simulink model "antrieb"  (Simulink 7.8)
settings: Solver=ode3  StartTime=0.0  StopTime=40  FixedStep=0.004  RelTol=1e-3
libraries: simulink x1
settings Model: Creator=Administrator  LastModifiedBy=antrieb  SimulationMode=external  ExtModeTrigDuration=500000  ExtModeTrigDurationFloating=300000
settings DataIOCC: LimitDataPoints=off  MaxDataPoints=100000  SaveFormat=StructureWithTime  SaveOutput=off  SignalLogging=off  SaveTime=off  SignalLoggingName=sigsOut
settings OptimizationCC: InitFltsAndDblsToZero=on
settings DebuggingCC: SaveWithParameterizedLinksMsg=none  SignalResolutionControl=TryResolveAllWithWarning  SolverPrmCheckMsg=none  MultiTaskDSMMsg=warning  MultiTaskCondExecSysMsg=none  FcnCallInpInsideContextMsg=Use local settings  StrictBusMsg=None
settings HardwareCC: TargetEndianess=LittleEndian  TargetHWDeviceType=MATLAB Host
settings RTWCC: SystemTargetFile=rtwin.tlc  TemplateMakefile=rtwin.tmf  Description=Real-Time Windows Target  ProcessScript=rtwin_make_rtw_hook  IncludeERTFirstTime=on
settings RTWinTargetCC: TargetFcnLib=ansi_tfl_tmw.mat  TargetLibSuffix=_rtwin.lib  TargetPreCompLibLocation=C:\Program Files\MATLAB\R2011b\toolbox\rtw\targets\rtwin\lib\win32  TargetFunctionLibrary=ANSI_C  CodeExecutionProfiling=off  ModelReferenceCompliant=off  CompOptLevelCompliant=off  PortableWordSizes=off  RTWinDir=C:/PROGRA~1/MATLAB/R2011b/toolbox/rtw/targets/rtwin  TargetArch=win32

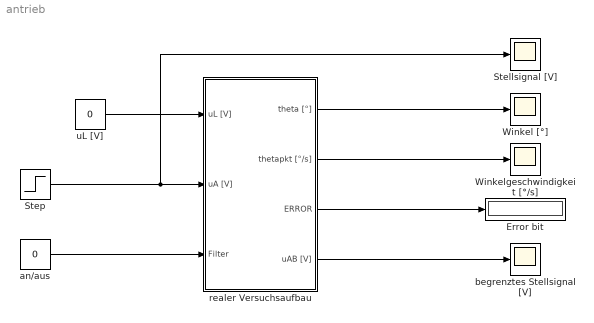
== system antrieb ==
  Error bit : Display
  Stellsignal [V] : Scope
      settings: TimeRange=40  YMin=0.95  YMax=1.05  SaveName=Stellsignal  MaxDataPoints=500000
  Step : Step  SampleTime=0
  Winkel [°] : Scope
      settings: TimeRange=40  YMin=0  YMax=10000  SaveName=Theta  MaxDataPoints=50000
  Winkelgeschwindigkeit [°/s] : Scope
      settings: TimeRange=40  YMin=0  YMax=2000  SaveName=Theta_pkt  MaxDataPoints=500000
  an/aus : Constant  Value=0
  begrenztes Stellsignal [V] : Scope
      settings: TimeRange=40  MaxDataPoints=500000
  realer Versuchsaufbau : Subsystem  mask{BaseAddr='0xD000', STime=0.004, TimeOutPer=500, HWAccess=on}
      mask prompts: BaseAddr "Base I/O Address"; STime "Sample Time [sec]"; TimeOutPer "Timeout Period (500 ~ 2000)"; HWAccess "Hardware Access"
  uL [V] : Constant  Value=0
  wires:
  realer Versuchsaufbau/3(ERROR) -> Error bit/1
  realer Versuchsaufbau/1(theta [°]) -> Winkel [°]/1
  realer Versuchsaufbau/2(thetapkt [°/s]) -> Winkelgeschwindigkeit [°/s]/1
  realer Versuchsaufbau/4(uAB [V]) -> begrenztes Stellsignal [V]/1
  uL [V]/1 -> realer Versuchsaufbau/1(uL [V])
  an/aus/1 -> realer Versuchsaufbau/3(Filter)
  Step/1 -> realer Versuchsaufbau/2(uA [V]), Stellsignal [V]/1

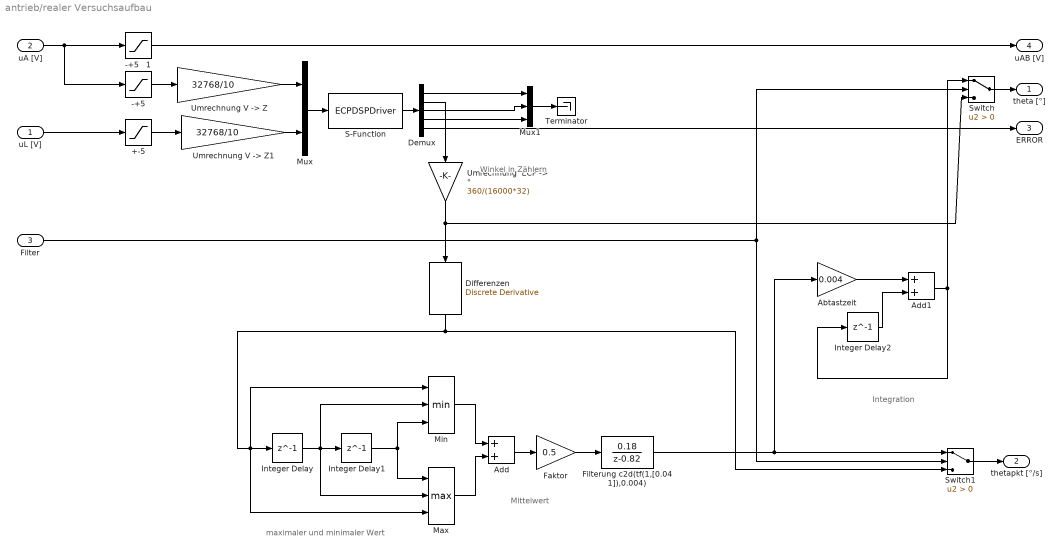
== system antrieb/realer Versuchsaufbau ==
  note: Winkel in Zählern
  note: maximaler und minimaler Wert
  note: Mittelwert
  note: Integration
  uL [V] : Inport
  uA [V] : Inport  Port=2
  Filter : Inport  Port=3
  "   +-5" : Saturate  UpperLimit=5  LowerLimit=-5
  "-+5   " : Saturate  UpperLimit=5  LowerLimit=-5
  -+5   1 : Saturate  UpperLimit=5  LowerLimit=-5
  Abtastzeit : Gain  Gain=0.004  SaturateOnIntegerOverflow=on  OutDataTypeStr=Inherit: Same as input  ParamDataTypeStr=Inherit: Same as input
  Add : Sum
  Add1 : Sum
  Demux : Demux  Outputs=5
  Differenzen : simulink/Discrete/Discrete Derivative  gainval=1.0  ICPrevScaledInput=0.0  InputProcessing=Inherited  OutMin=[]  OutMax=[]  OutDataType=sfix(16)  OutScaling=2^-10  DoSatur=off
  Faktor : Gain  Gain=0.5  SaturateOnIntegerOverflow=on  OutDataTypeStr=Inherit: Same as input  ParamDataTypeStr=Inherit: Same as input
  Filterung c2d(tf(1,[0.04 1]),0.004) : DiscreteTransferFcn  Numerator=0.18  Denominator=[1 -0.82]  SampleTime=-1
  Integer Delay : Delay  DelayLength=1  InputProcessing=Inherited
  Integer Delay1 : Delay  DelayLength=1  InputProcessing=Inherited
  Integer Delay2 : Delay  DelayLength=1  InputProcessing=Inherited
  Max : MinMax  Function=max  Inputs=3
  Min : MinMax  Inputs=3
  Mux : Mux  Inputs=2
  Mux1 : Mux  Inputs=3
  S-Function : S-Function  FunctionName=ECPDSPDriver  Parameters=BaseAddr,STime,TimeOutPer,HWAccess  EnableBusSupport=off
  Switch : Switch  Criteria=u2 > Threshold
  Switch1 : Switch  Criteria=u2 > Threshold
  Terminator : Terminator
  "Umrechnung  ECP -> °" : Gain  Gain=360/(16000*32)  SaturateOnIntegerOverflow=on  OutDataTypeStr=Inherit: Same as input  ParamDataTypeStr=Inherit: Same as input
  "Umrechnung V -> Z" : Gain  Gain=32768/10  SaturateOnIntegerOverflow=on  OutDataTypeStr=Inherit: Same as input  ParamDataTypeStr=Inherit: Same as input
  "Umrechnung V -> Z1" : Gain  Gain=32768/10  SaturateOnIntegerOverflow=on  OutDataTypeStr=Inherit: Same as input  ParamDataTypeStr=Inherit: Same as input
  theta [°] : Outport
  thetapkt [°/s] : Outport  Port=2
  ERROR : Outport  Port=3
  uAB [V] : Outport  Port=4
  wires:
  "-+5   "/1 -> "Umrechnung V -> Z"/1
  Mux/1 -> S-Function/1
  "Umrechnung V -> Z"/1 -> Mux/1
  "   +-5"/1 -> "Umrechnung V -> Z1"/1
  "Umrechnung V -> Z1"/1 -> Mux/2
  S-Function/1 -> Demux/1
  Mux1/1 -> Terminator/1
  Demux/1 -> Mux1/1
  Demux/3 -> Mux1/2
  Demux/4 -> Mux1/3
  uA [V]/1 -> -+5   1/1, "-+5   "/1
  uL [V]/1 -> "   +-5"/1
  Demux/5 -> ERROR/1
  Integer Delay/1 -> Min/2, Integer Delay1/1, Max/2
  Integer Delay1/1 -> Min/3, Max/1
  Min/1 -> Add/1
  Max/1 -> Add/2
  Add/1 -> Faktor/1
  Faktor/1 -> Filterung c2d(tf(1,[0.04 1]),0.004)/1
  Integer Delay2/1 -> Add1/2
  Add1/1 -> Integer Delay2/1, Switch/1
  Abtastzeit/1 -> Add1/1
  Filterung c2d(tf(1,[0.04 1]),0.004)/1 -> Abtastzeit/1, Switch1/1
  Demux/2 -> "Umrechnung  ECP -> °"/1
  Switch/1 -> theta [°]/1
  Filter/1 -> Switch/2, Switch1/2
  Switch1/1 -> thetapkt [°/s]/1
  "Umrechnung  ECP -> °"/1 -> Switch/3, Differenzen/1
  -+5   1/1 -> uAB [V]/1
  Differenzen/1 -> Integer Delay/1, Min/1, Max/3, Switch1/3
